simulink model "arm_sim_AC"  (R2013a)
settings: Solver=ode45  StartTime=0.0  StopTime=100  RelTol=1e-3
undefined symbols (not defined in the file or in its folder): arm_ctrl2, drawArm
settings Model: Creator=beard  LastModifiedBy=daqing_yi
settings DataIOCC: SignalLoggingSaveFormat=ModelDataLogs
settings OptimizationCC: ExpressionDepthLimit=2147483647  InitFltsAndDblsToZero=on
settings DebuggingCC: MultiTaskDSMMsg=warning  MultiTaskCondExecSysMsg=none  FcnCallInpInsideContextMsg=UseLocalSettings  StrictBusMsg=None
settings RTWCC: IncludeERTFirstTime=on
settings GRTTargetCC: CombineOutputUpdateFcns=off  GRTInterface=on

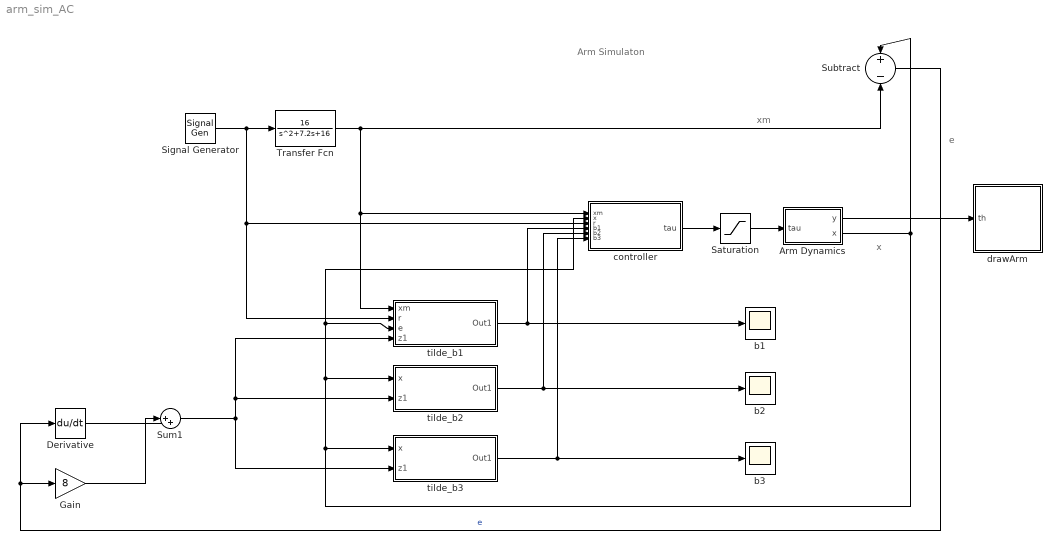
== system arm_sim_AC ==
  note: e
  note: x
  note: xm
  note: Arm Simulaton
  Arm Dynamics : Subsystem
  Derivative : Derivative
  Gain : Gain  Gain=8
  Saturation : Saturate  UpperLimit=2  LowerLimit=-2
  Signal Generator : SignalGenerator  WaveForm=square  Amplitude=25*pi/180  Frequency=.05
  Subtract : Sum  Inputs=+-
  Sum1 : Sum  Inputs=|++
  Transfer Fcn : TransferFcn  Numerator=[16]  Denominator=[1 7.2 16]
  b1 : Scope
      settings: YMin=0  YMax=1.2e+07
  b2 : Scope
      settings: YMin=0.95  YMax=1.05  SaveName=ScopeData3
  b3 : Scope
      settings: SaveName=ScopeData4
  controller : Subsystem
  drawArm : Subsystem
      mask init:
      | % drawing parameters
      | L = 1;
      | w = 0.3;
      mask Display: image(imread('tv.jpg'))
  tilde_b1 : Subsystem
  tilde_b2 : Subsystem
  tilde_b3 : Subsystem
  wires:
  controller/1(tau) -> Saturation/1
  Saturation/1 -> Arm Dynamics/1(tau)
  Arm Dynamics/1(y) -> drawArm/1(th)
  tilde_b1/1(Out1) -> b1/1, controller/4(b1)
  tilde_b2/1(Out1) -> controller/5(b2), b2/1
  tilde_b3/1(Out1) -> controller/6(b3), b3/1
  Signal Generator/1 -> tilde_b1/2(r), controller/3(r), Transfer Fcn/1
  Subtract/1 -> Derivative/1, Gain/1  "e"
  Gain/1 -> Sum1/1
  Derivative/1 -> Sum1/2
  Sum1/1 -> tilde_b2/2(z1), tilde_b1/4(z1), tilde_b3/2(z1)
  Arm Dynamics/2(x) -> tilde_b3/1(x), tilde_b2/1("x "), controller/2(x), tilde_b1/3(e), Subtract/1
  Transfer Fcn/1 -> tilde_b1/1(xm), controller/1(xm), Subtract/2

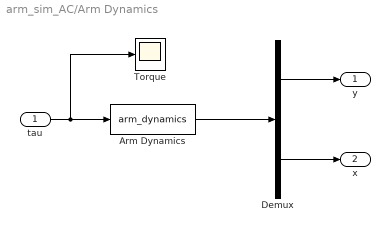
== system arm_sim_AC/Arm Dynamics ==
  tau : Inport
  Arm Dynamics : S-Function  FunctionName=arm_dynamics  EnableBusSupport=off
  Demux : Demux  Outputs=[1;2]
  Torque : Scope
      settings: TimeRange=100  YMin=-1  YMax=2  SaveName=ScopeData2
  y : Outport
  x : Outport  Port=2
  wires:
  tau/1 -> Arm Dynamics/1, Torque/1
  Arm Dynamics/1 -> Demux/1
  Demux/1 -> y/1
  Demux/2 -> x/1

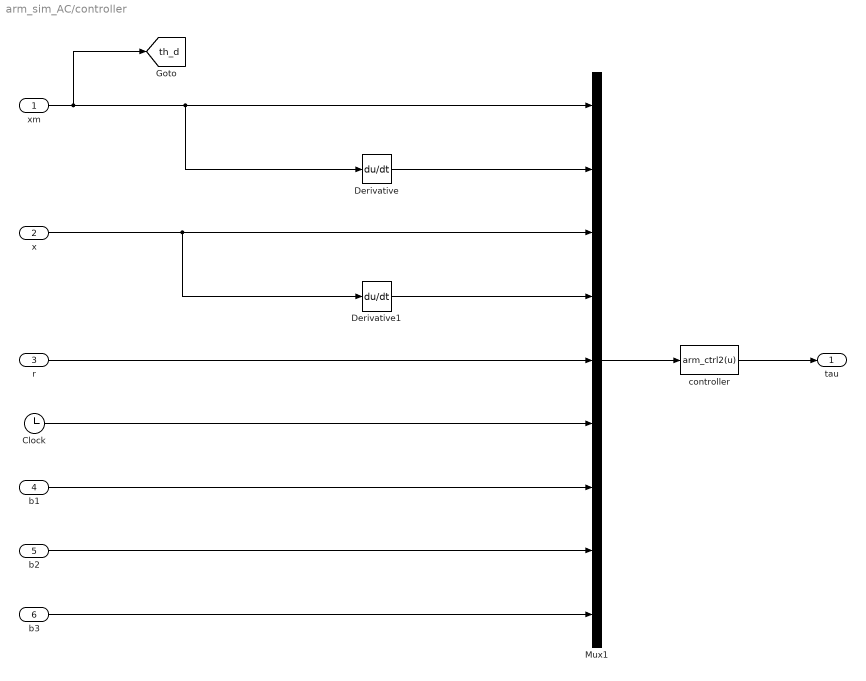
== system arm_sim_AC/controller ==
  xm : Inport
  x : Inport  Port=2
  r : Inport  Port=3
  b1 : Inport  Port=4
  b2 : Inport  Port=5
  b3 : Inport  Port=6
  Clock : Clock
  Derivative : Derivative
  Derivative1 : Derivative
  Mux1 : Mux  Inputs=9
  controller : MATLABFcn  MATLABFcn=arm_ctrl2(u)  OutputDimensions=1  SampleTime=0.01
  tau : Outport
  tag scope: th_d=global
  wires:
  Mux1/1 -> controller/1
  controller/1 -> tau/1
  b2/1 -> Mux1/8
  xm/1 -> [th_d], Derivative/1, Mux1/1
  b1/1 -> Mux1/7
  Clock/1 -> Mux1/6
  b3/1 -> Mux1/9
  Derivative/1 -> Mux1/2
  x/1 -> Derivative1/1, Mux1/3
  Derivative1/1 -> Mux1/4
  r/1 -> Mux1/5

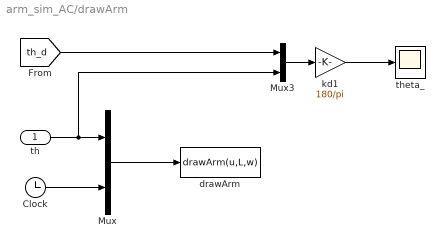
== system arm_sim_AC/drawArm ==
  th : Inport
  Clock : Clock
  Mux : Mux  Inputs=2
  Mux3 : Mux  Inputs=2
  drawArm : MATLABFcn  MATLABFcn=drawArm(u,L,w)  OutputDimensions=0  SampleTime=0.1
  kd1 : Gain  Gain=180/pi
  theta_ : Scope
      settings: TimeRange=100  YMin=-27.5  YMax=27.5
  wires:
  Mux/1 -> drawArm/1
  th/1 -> Mux3/2, Mux/1
  Clock/1 -> Mux/2
  [th_d] -> Mux3/1
  Mux3/1 -> kd1/1
  kd1/1 -> theta_/1

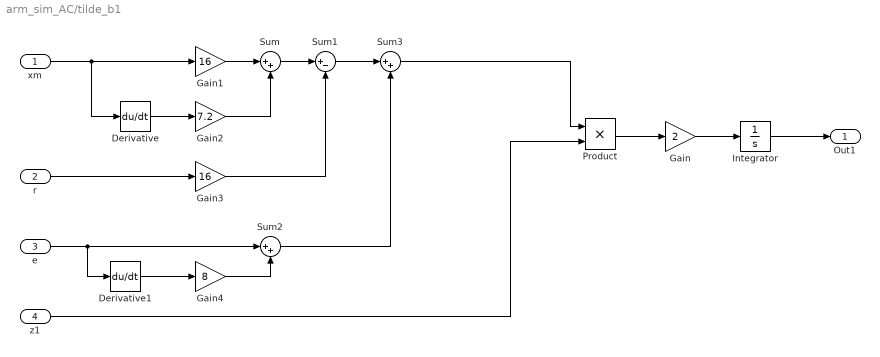
== system arm_sim_AC/tilde_b1 ==
  xm : Inport
  r : Inport  Port=2
  e : Inport  Port=3
  z1 : Inport  Port=4
  Derivative : Derivative
  Derivative1 : Derivative
  Gain : Gain  Gain=2
  Gain1 : Gain  Gain=16
  Gain2 : Gain  Gain=7.2
  Gain3 : Gain  Gain=16
  Gain4 : Gain  Gain=8
  Integrator : Integrator  InitialCondition=0.2
  Product : Product
  Sum : Sum  Inputs=|++
  Sum1 : Sum  Inputs=|+-
  Sum2 : Sum  Inputs=|++
  Sum3 : Sum  Inputs=|++
  Out1 : Outport
  wires:
  Integrator/1 -> Out1/1
  Gain/1 -> Integrator/1
  xm/1 -> Derivative/1, Gain1/1
  Derivative/1 -> Gain2/1
  r/1 -> Gain3/1
  Product/1 -> Gain/1
  z1/1 -> Product/2
  Gain1/1 -> Sum/1
  Gain2/1 -> Sum/2
  Sum/1 -> Sum1/1
  Gain3/1 -> Sum1/2
  Derivative1/1 -> Gain4/1
  e/1 -> Derivative1/1, Sum2/1
  Gain4/1 -> Sum2/2
  Sum1/1 -> Sum3/1
  Sum2/1 -> Sum3/2
  Sum3/1 -> Product/1

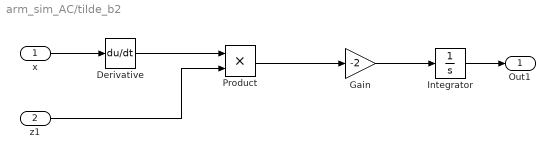
== system arm_sim_AC/tilde_b2 ==
  "x " : Inport
  z1 : Inport  Port=2
  Derivative : Derivative
  Gain : Gain  Gain=-2
  Integrator : Integrator  InitialCondition=0.1
  Product : Product
  Out1 : Outport
  wires:
  Integrator/1 -> Out1/1
  "x "/1 -> Derivative/1
  Gain/1 -> Integrator/1
  Derivative/1 -> Product/1
  z1/1 -> Product/2
  Product/1 -> Gain/1

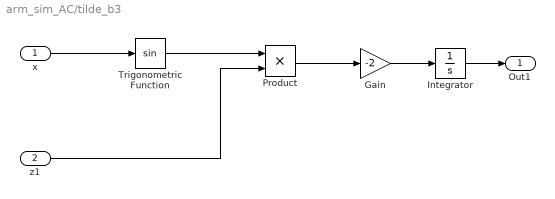
== system arm_sim_AC/tilde_b3 ==
  x : Inport
  z1 : Inport  Port=2
  Gain : Gain  Gain=-2
  Integrator : Integrator  InitialCondition=0.1
  Product : Product
  Trigonometric Function : Trigonometry
  Out1 : Outport
  wires:
  Integrator/1 -> Out1/1
  x/1 -> Trigonometric Function/1
  Gain/1 -> Integrator/1
  Product/1 -> Gain/1
  Trigonometric Function/1 -> Product/1
  z1/1 -> Product/2
